simulink library "halout"  (R2021b)
settings: Solver=VariableStepAuto  StartTime=0.0  StopTime=10.0  RelTol=1e-3
undefined symbols (not defined in the file): C_TASK_5MS_S, FALSE, KHAL_CAN1FDAPS3E2E_flg, KHAL_CAN1FDAPS3TxReq_flg, KHAL_CAN1FDVCU2E2E_flg, KHAL_CAN1FDVCU2TxReq_flg, KHAL_CAN1FDVCU3E2E_flg, KHAL_CAN1FDVCU3TxReq_flg, KHAL_CAN1TxReq_flg, KHAL_CAN2TxReq_flg, KHAL_CAN3FDVCU1TxReq_flg, KHAL_CAN3FDVCU2E2E_flg, KHAL_CAN3FDVCU2TxReq_flg, KHAL_CAN3TxReq_flg, KHAL_CAN4FDVCU1E2E_flg, KHAL_CAN4FDVCU1TxReq_flg, KHAL_CAN4TxReq_flg, KHAL_CAN5TxReq_flg, ONE_INT, TRUE, ZERO_INT
libraries: FVT_lib x383, simulink x179
(part 8 of 20)

== system halout/HAL_OUT/CAN4/FD_DKC1_0x253 ==
  BSCP_outputs : Inport  OutDataTypeStr=Bus: BSCP_outputs
  BOUTP_outputs : Inport  Port=2  OutDataTypeStr=Bus: BOUTP_outputs
  ApproachUnlockSW : Subsystem
  BrkPedalPos : Subsystem
  BrkPedalPosSta : Subsystem
  BrkSwSta : Subsystem
  BrkSwV : Subsystem
  DSEATantiset : Subsystem
  DSEATentryfunset : Subsystem
  DSEATventreq : Subsystem
  FDCBCMATCtrlCmd : Subsystem
  FDCBCMLockAlarmCmd : Subsystem
  FDCBCMOutModeCmd : Subsystem
  FDCTHCMACTInitialCmd : Subsystem
  Ground1 : Ground
  HeadLampSW : Subsystem
  HoodLatchSW : Subsystem
  IVIISAOffsetSpd : Subsystem
  IVILocatedSTA : Subsystem
  IVIPTGModeSW : Subsystem
  IVIPTGOpenHeight : Subsystem
  IVIPTGStaSW : Subsystem
  IVIPTGUSStaSW : Subsystem
  IVITimeCheck : Subsystem
  IVITimeDay : Subsystem
  IVITimeHour : Subsystem
  IVITimeMinute : Subsystem
  IVITimeMonth : Subsystem
  IVITimeSecond : Subsystem
  IVITimeYear : Subsystem
  LDrvCtrlCmd : Subsystem
  LPasCtrlCmd : Subsystem
  LRLDCtrlCmd : Subsystem
  LRRDCtrlCmd : Subsystem
  MCPressure : Subsystem
  MCPressureV : Subsystem
  OFFACMODE : Subsystem
  PSEATventreq : Subsystem
  PTGInnerSW2 : Subsystem
  SenstivityPosition : Subsystem
  TurnSwTimeSet : Subsystem
  WalkawayLockSW : Subsystem
  bus_creator : BusCreator  Inputs=39  OutDataTypeStr=Bus: DT_CAN4_SG_FD_DKC1  NonVirtualBus=on
  bus_selector : BusSelector  OutputSignals=VSCP_CAN4FDDKC1ApproachUnlockSW_flg
  bus_selector1 : BusSelector  OutputSignals=VSCP_CAN4FDDKC1BrkPedalPos_pct
  bus_selector10 : BusSelector  OutputSignals=VSCP_CAN4FDDKC1HeadLampSW_enum
  bus_selector11 : BusSelector  OutputSignals=VSCP_CAN4FDDKC1HoodLatchSW_enum
  bus_selector12 : BusSelector  OutputSignals=VSCP_CAN4FDDKC1IVIISAOffsetSpd_enum
  bus_selector13 : BusSelector  OutputSignals=VSCP_CAN4FDDKC1IVILocatedSTA_enum
  bus_selector14 : BusSelector  OutputSignals=VSCP_CAN4FDDKC1IVIPTGModeSW_enum
  bus_selector15 : BusSelector  OutputSignals=VSCP_CAN4FDDKC1IVIPTGOpenHeight_enum
  bus_selector16 : BusSelector  OutputSignals=VSCP_CAN4FDDKC1IVIPTGStaSW_enum
  bus_selector17 : BusSelector  OutputSignals=VSCP_CAN4FDDKC1IVIPTGUSStaSW_flg
  bus_selector18 : BusSelector  OutputSignals=VSCP_CAN4FDDKC1IVITimeCheck_enum
  bus_selector19 : BusSelector  OutputSignals=VSCP_CAN4FDDKC1IVITimeDay_DAY
  bus_selector2 : BusSelector  OutputSignals=VSCP_CAN4FDDKC1BrkPedalPosSta_flg
  bus_selector20 : BusSelector  OutputSignals=VSCP_CAN4FDDKC1IVITimeHour_hr
  bus_selector21 : BusSelector  OutputSignals=VSCP_CAN4FDDKC1IVITimeMinute_min
  bus_selector22 : BusSelector  OutputSignals=VSCP_CAN4FDDKC1IVITimeMonth_MONTH
  bus_selector23 : BusSelector  OutputSignals=VSCP_CAN4FDDKC1IVITimeSecond_s
  bus_selector24 : BusSelector  OutputSignals=VSCP_CAN4FDDKC1IVITimeYear_YEAR
  bus_selector25 : BusSelector  OutputSignals=VOUTP_LDrvCtrlCmd_pct
  bus_selector26 : BusSelector  OutputSignals=VOUTP_LPasCtrlCmd_pct
  bus_selector27 : BusSelector  OutputSignals=VOUTP_LRLDCtrlCmd_pct
  bus_selector28 : BusSelector  OutputSignals=VOUTP_LRRDCtrlCmd_pct
  bus_selector29 : BusSelector  OutputSignals=VSCP_CAN4FDDKC1MCPressure_bar
  bus_selector3 : BusSelector  OutputSignals=VSCP_CAN4FDDKC1BrkSwSta_flg
  bus_selector30 : BusSelector  OutputSignals=VSCP_CAN4FDDKC1MCPressureV_flg
  bus_selector31 : BusSelector  OutputSignals=VSCP_CAN4FDDKC1OFFACMODE_enum
  bus_selector32 : BusSelector  OutputSignals=VSCP_CAN4FDDKC1PSEATventreq_enum
  bus_selector33 : BusSelector  OutputSignals=VOUTP_PTGInnerSW2_enum
  bus_selector34 : BusSelector  OutputSignals=VSCP_CAN4FDDKC1SenstivityPosition_enum
  bus_selector35 : BusSelector  OutputSignals=VSCP_CAN4FDDKC1TurnSwTimeSet_enum
  bus_selector36 : BusSelector  OutputSignals=VSCP_CAN4FDDKC1WalkawayLockSW_flg
  bus_selector37 : BusSelector  OutputSignals=VOUTP_OutMode_enum
  bus_selector4 : BusSelector  OutputSignals=VSCP_CAN4FDDKC1BrkSwV_flg
  bus_selector5 : BusSelector  OutputSignals=VSCP_CAN4FDDKC1DSEATantiset_flg
  bus_selector6 : BusSelector  OutputSignals=VSCP_CAN4FDDKC1DSEATentryfunset_flg
  bus_selector7 : BusSelector  OutputSignals=VSCP_CAN4FDDKC1DSEATventreq_enum
  bus_selector8 : BusSelector  OutputSignals=VOUTP_ATCtrl_enum
  bus_selector9 : BusSelector  OutputSignals=VOUTP_LockAlarm_enum
  FD_DKC1 : Outport
  wires:
  BSCP_outputs/1 -> [BSCP_outputs]
  BOUTP_outputs/1 -> [BOUTP_outputs]
  [CAN4_Approach_Unlock_SW] -> bus_creator/1  "CAN4_Approach_Unlock_SW"
  [CAN4_BrkPedalPos] -> bus_creator/2  "CAN4_BrkPedalPos"
  [CAN4_BrkPedalPos_Sta] -> bus_creator/3  "CAN4_BrkPedalPos_Sta"
  [CAN4_BrkSw_Sta] -> bus_creator/4  "CAN4_BrkSw_Sta"
  [CAN4_BrkSw_V] -> bus_creator/5  "CAN4_BrkSw_V"
  [CAN4_DSEAT_anti_set] -> bus_creator/6  "CAN4_DSEAT_anti_set"
  [CAN4_DSEAT_entryfun_set] -> bus_creator/7  "CAN4_DSEAT_entryfun_set"
  [CAN4_DSEAT_vent_req] -> bus_creator/8  "CAN4_DSEAT_vent_req"
  [CAN4_FDC_BCM_ATCtrl_Cmd] -> bus_creator/9  "CAN4_FDC_BCM_ATCtrl_Cmd"
  [CAN4_FDC_BCM_LockAlarm_Cmd] -> bus_creator/10  "CAN4_FDC_BCM_LockAlarm_Cmd"
  [CAN4_FDC_BCM_OutMode_Cmd] -> bus_creator/11  "CAN4_FDC_BCM_OutMode_Cmd"
  [CAN4_FDC_THCM_ACTInitial_Cmd] -> bus_creator/12  "CAN4_FDC_THCM_ACTInitial_Cmd"
  [CAN4_HeadLampSW] -> bus_creator/13  "CAN4_HeadLampSW"
  [CAN4_Hood_Latch_SW] -> bus_creator/14  "CAN4_Hood_Latch_SW"
  [CAN4_IVI_ISA_OffsetSpd] -> bus_creator/15  "CAN4_IVI_ISA_OffsetSpd"
  [CAN4_IVI_Located_STA] -> bus_creator/16  "CAN4_IVI_Located_STA"
  [CAN4_IVI_PTG_Mode_SW] -> bus_creator/17  "CAN4_IVI_PTG_Mode_SW"
  [CAN4_IVI_PTG_Open_Height] -> bus_creator/18  "CAN4_IVI_PTG_Open_Height"
  [CAN4_IVI_PTG_Sta_SW] -> bus_creator/19  "CAN4_IVI_PTG_Sta_SW"
  [CAN4_IVI_PTG_USSta_SW] -> bus_creator/20  "CAN4_IVI_PTG_USSta_SW"
  [CAN4_IVI_Time_Check] -> bus_creator/21  "CAN4_IVI_Time_Check"
  [CAN4_IVI_Time_Day] -> bus_creator/22  "CAN4_IVI_Time_Day"
  [CAN4_IVI_Time_Hour] -> bus_creator/23  "CAN4_IVI_Time_Hour"
  [CAN4_IVI_Time_Minute] -> bus_creator/24  "CAN4_IVI_Time_Minute"
  [CAN4_IVI_Time_Month] -> bus_creator/25  "CAN4_IVI_Time_Month"
  [CAN4_IVI_Time_Second] -> bus_creator/26  "CAN4_IVI_Time_Second"
  [CAN4_IVI_Time_Year] -> bus_creator/27  "CAN4_IVI_Time_Year"
  [CAN4_L_Drv_CtrlCmd] -> bus_creator/28  "CAN4_L_Drv_CtrlCmd"
  [CAN4_L_Pas_CtrlCmd] -> bus_creator/29  "CAN4_L_Pas_CtrlCmd"
  [CAN4_L_RLD_CtrlCmd] -> bus_creator/30  "CAN4_L_RLD_CtrlCmd"
  [CAN4_L_RRD_CtrlCmd] -> bus_creator/31  "CAN4_L_RRD_CtrlCmd"
  [CAN4_MCPressure] -> bus_creator/32  "CAN4_MCPressure"
  [CAN4_MCPressure_V] -> bus_creator/33  "CAN4_MCPressure_V"
  [CAN4_OFF_AC_MODE] -> bus_creator/34  "CAN4_OFF_AC_MODE"
  [CAN4_PSEAT_vent_req] -> bus_creator/35  "CAN4_PSEAT_vent_req"
  [CAN4_PTG_Inner_SW2] -> bus_creator/36  "CAN4_PTG_Inner_SW2"
  [CAN4_SenstivityPosition] -> bus_creator/37  "CAN4_SenstivityPosition"
  [CAN4_TurnSwTimeSet] -> bus_creator/38  "CAN4_TurnSwTimeSet"
  [CAN4_Walkaway_Lock_SW] -> bus_creator/39  "CAN4_Walkaway_Lock_SW"
  bus_creator/1 -> FD_DKC1/1
  ApproachUnlockSW/1(CAN4_Approach_Unlock_SW) -> [CAN4_Approach_Unlock_SW]
  BrkPedalPos/1(CAN4_BrkPedalPos) -> [CAN4_BrkPedalPos]
  BrkPedalPosSta/1(CAN4_BrkPedalPos_Sta) -> [CAN4_BrkPedalPos_Sta]
  BrkSwSta/1(CAN4_BrkSw_Sta) -> [CAN4_BrkSw_Sta]
  BrkSwV/1(CAN4_BrkSw_V) -> [CAN4_BrkSw_V]
  DSEATantiset/1(CAN4_DSEAT_anti_set) -> [CAN4_DSEAT_anti_set]
  DSEATentryfunset/1(CAN4_DSEAT_entryfun_set) -> [CAN4_DSEAT_entryfun_set]
  DSEATventreq/1(CAN4_DSEAT_vent_req) -> [CAN4_DSEAT_vent_req]
  FDCBCMATCtrlCmd/1(CAN4_FDC_BCM_ATCtrl_Cmd) -> [CAN4_FDC_BCM_ATCtrl_Cmd]
  FDCBCMLockAlarmCmd/1(CAN4_FDC_BCM_LockAlarm_Cmd) -> [CAN4_FDC_BCM_LockAlarm_Cmd]
  FDCBCMOutModeCmd/1(CAN4_FDC_BCM_OutMode_Cmd) -> [CAN4_FDC_BCM_OutMode_Cmd]
  FDCTHCMACTInitialCmd/1(CAN4_FDC_THCM_ACTInitial_Cmd) -> [CAN4_FDC_THCM_ACTInitial_Cmd]
  HeadLampSW/1(CAN4_HeadLampSW) -> [CAN4_HeadLampSW]
  HoodLatchSW/1(CAN4_Hood_Latch_SW) -> [CAN4_Hood_Latch_SW]
  IVIISAOffsetSpd/1(CAN4_IVI_ISA_OffsetSpd) -> [CAN4_IVI_ISA_OffsetSpd]
  IVILocatedSTA/1(CAN4_IVI_Located_STA) -> [CAN4_IVI_Located_STA]
  IVIPTGModeSW/1(CAN4_IVI_PTG_Mode_SW) -> [CAN4_IVI_PTG_Mode_SW]
  IVIPTGOpenHeight/1(CAN4_IVI_PTG_Open_Height) -> [CAN4_IVI_PTG_Open_Height]
  IVIPTGStaSW/1(CAN4_IVI_PTG_Sta_SW) -> [CAN4_IVI_PTG_Sta_SW]
  IVIPTGUSStaSW/1(CAN4_IVI_PTG_USSta_SW) -> [CAN4_IVI_PTG_USSta_SW]
  IVITimeCheck/1(CAN4_IVI_Time_Check) -> [CAN4_IVI_Time_Check]
  IVITimeDay/1(CAN4_IVI_Time_Day) -> [CAN4_IVI_Time_Day]
  IVITimeHour/1(CAN4_IVI_Time_Hour) -> [CAN4_IVI_Time_Hour]
  IVITimeMinute/1(CAN4_IVI_Time_Minute) -> [CAN4_IVI_Time_Minute]
  IVITimeMonth/1(CAN4_IVI_Time_Month) -> [CAN4_IVI_Time_Month]
  IVITimeSecond/1(CAN4_IVI_Time_Second) -> [CAN4_IVI_Time_Second]
  IVITimeYear/1(CAN4_IVI_Time_Year) -> [CAN4_IVI_Time_Year]
  LDrvCtrlCmd/1(CAN4_L_Drv_CtrlCmd) -> [CAN4_L_Drv_CtrlCmd]
  LPasCtrlCmd/1(CAN4_L_Pas_CtrlCmd) -> [CAN4_L_Pas_CtrlCmd]
  LRLDCtrlCmd/1(CAN4_L_RLD_CtrlCmd) -> [CAN4_L_RLD_CtrlCmd]
  LRRDCtrlCmd/1(CAN4_L_RRD_CtrlCmd) -> [CAN4_L_RRD_CtrlCmd]
  MCPressure/1(CAN4_MCPressure) -> [CAN4_MCPressure]
  MCPressureV/1(CAN4_MCPressure_V) -> [CAN4_MCPressure_V]
  OFFACMODE/1(CAN4_OFF_AC_MODE) -> [CAN4_OFF_AC_MODE]
  PSEATventreq/1(CAN4_PSEAT_vent_req) -> [CAN4_PSEAT_vent_req]
  PTGInnerSW2/1(CAN4_PTG_Inner_SW2) -> [CAN4_PTG_Inner_SW2]
  SenstivityPosition/1(CAN4_SenstivityPosition) -> [CAN4_SenstivityPosition]
  TurnSwTimeSet/1(CAN4_TurnSwTimeSet) -> [CAN4_TurnSwTimeSet]
  WalkawayLockSW/1(CAN4_Walkaway_Lock_SW) -> [CAN4_Walkaway_Lock_SW]
  bus_selector/1 -> ApproachUnlockSW/1(ApproachUnlockSW)  "<VSCP_CAN4FDDKC1ApproachUnlockSW_flg>"
  [BSCP_outputs] -> bus_selector/1
  bus_selector1/1 -> BrkPedalPos/1(BrkPedalPos)  "<VSCP_CAN4FDDKC1BrkPedalPos_pct>"
  [BSCP_outputs] -> bus_selector1/1
  bus_selector2/1 -> BrkPedalPosSta/1(BrkPedalPosSta)  "<VSCP_CAN4FDDKC1BrkPedalPosSta_flg>"
  [BSCP_outputs] -> bus_selector2/1
  bus_selector3/1 -> BrkSwSta/1(BrkSwSta)  "<VSCP_CAN4FDDKC1BrkSwSta_flg>"
  [BSCP_outputs] -> bus_selector3/1
  bus_selector4/1 -> BrkSwV/1(BrkSwV)  "<VSCP_CAN4FDDKC1BrkSwV_flg>"
  [BSCP_outputs] -> bus_selector4/1
  bus_selector5/1 -> DSEATantiset/1(DSEATantiset)  "<VSCP_CAN4FDDKC1DSEATantiset_flg>"
  [BSCP_outputs] -> bus_selector5/1
  bus_selector6/1 -> DSEATentryfunset/1(DSEATentryfunset)  "<VSCP_CAN4FDDKC1DSEATentryfunset_flg>"
  [BSCP_outputs] -> bus_selector6/1
  bus_selector7/1 -> DSEATventreq/1(DSEATventreq)  "<VSCP_CAN4FDDKC1DSEATventreq_enum>"
  [BSCP_outputs] -> bus_selector7/1
  bus_selector8/1 -> FDCBCMATCtrlCmd/1(FDCBCMATCtrlCmd)  "<VOUTP_ATCtrl_enum>"
  [BOUTP_outputs] -> bus_selector8/1
  bus_selector9/1 -> FDCBCMLockAlarmCmd/1(FDCBCMLockAlarmCmd)  "<VOUTP_LockAlarm_enum>"
  [BOUTP_outputs] -> bus_selector9/1
  Ground1/1 -> FDCTHCMACTInitialCmd/1(FDCTHCMACTInitialCmd)
  bus_selector10/1 -> HeadLampSW/1(HeadLampSW)  "<VSCP_CAN4FDDKC1HeadLampSW_enum>"
  [BSCP_outputs] -> bus_selector10/1
  bus_selector11/1 -> HoodLatchSW/1(HoodLatchSW)  "<VSCP_CAN4FDDKC1HoodLatchSW_enum>"
  [BSCP_outputs] -> bus_selector11/1
  bus_selector12/1 -> IVIISAOffsetSpd/1(IVIISAOffsetSpd)  "<VSCP_CAN4FDDKC1IVIISAOffsetSpd_enum>"
  [BSCP_outputs] -> bus_selector12/1
  bus_selector13/1 -> IVILocatedSTA/1(IVILocatedSTA)  "<VSCP_CAN4FDDKC1IVILocatedSTA_enum>"
  [BSCP_outputs] -> bus_selector13/1
  bus_selector14/1 -> IVIPTGModeSW/1(IVIPTGModeSW)  "<VSCP_CAN4FDDKC1IVIPTGModeSW_enum>"
  [BSCP_outputs] -> bus_selector14/1
  bus_selector15/1 -> IVIPTGOpenHeight/1(IVIPTGOpenHeight)  "<VSCP_CAN4FDDKC1IVIPTGOpenHeight_enum>"
  [BSCP_outputs] -> bus_selector15/1
  bus_selector16/1 -> IVIPTGStaSW/1(IVIPTGStaSW)  "<VSCP_CAN4FDDKC1IVIPTGStaSW_enum>"
  [BSCP_outputs] -> bus_selector16/1
  bus_selector17/1 -> IVIPTGUSStaSW/1(IVIPTGUSStaSW)  "<VSCP_CAN4FDDKC1IVIPTGUSStaSW_flg>"
  [BSCP_outputs] -> bus_selector17/1
  bus_selector18/1 -> IVITimeCheck/1(IVITimeCheck)  "<VSCP_CAN4FDDKC1IVITimeCheck_enum>"
  [BSCP_outputs] -> bus_selector18/1
  bus_selector19/1 -> IVITimeDay/1(IVITimeDay)  "<VSCP_CAN4FDDKC1IVITimeDay_DAY>"
  [BSCP_outputs] -> bus_selector19/1
  bus_selector20/1 -> IVITimeHour/1(IVITimeHour)  "<VSCP_CAN4FDDKC1IVITimeHour_hr>"
  [BSCP_outputs] -> bus_selector20/1
  bus_selector21/1 -> IVITimeMinute/1(IVITimeMinute)  "<VSCP_CAN4FDDKC1IVITimeMinute_min>"
  [BSCP_outputs] -> bus_selector21/1
  bus_selector22/1 -> IVITimeMonth/1(IVITimeMonth)  "<VSCP_CAN4FDDKC1IVITimeMonth_MONTH>"
  [BSCP_outputs] -> bus_selector22/1
  bus_selector23/1 -> IVITimeSecond/1(IVITimeSecond)  "<VSCP_CAN4FDDKC1IVITimeSecond_s>"
  [BSCP_outputs] -> bus_selector23/1
  bus_selector24/1 -> IVITimeYear/1(IVITimeYear)  "<VSCP_CAN4FDDKC1IVITimeYear_YEAR>"
  [BSCP_outputs] -> bus_selector24/1
  bus_selector25/1 -> LDrvCtrlCmd/1(LDrvCtrlCmd)  "<VOUTP_LDrvCtrlCmd_pct>"
  [BOUTP_outputs] -> bus_selector25/1
  bus_selector26/1 -> LPasCtrlCmd/1(LPasCtrlCmd)  "<VOUTP_LPasCtrlCmd_pct>"
  [BOUTP_outputs] -> bus_selector26/1
  bus_selector27/1 -> LRLDCtrlCmd/1(LRLDCtrlCmd)  "<VOUTP_LRLDCtrlCmd_pct>"
  [BOUTP_outputs] -> bus_selector27/1
  bus_selector28/1 -> LRRDCtrlCmd/1(LRRDCtrlCmd)  "<VOUTP_LRRDCtrlCmd_pct>"
  [BOUTP_outputs] -> bus_selector28/1
  bus_selector29/1 -> MCPressure/1(MCPressure)  "<VSCP_CAN4FDDKC1MCPressure_bar>"
  [BSCP_outputs] -> bus_selector29/1
  bus_selector30/1 -> MCPressureV/1(MCPressureV)  "<VSCP_CAN4FDDKC1MCPressureV_flg>"
  [BSCP_outputs] -> bus_selector30/1
  bus_selector31/1 -> OFFACMODE/1(OFFACMODE)  "<VSCP_CAN4FDDKC1OFFACMODE_enum>"
  [BSCP_outputs] -> bus_selector31/1
  bus_selector32/1 -> PSEATventreq/1(PSEATventreq)  "<VSCP_CAN4FDDKC1PSEATventreq_enum>"
  [BSCP_outputs] -> bus_selector32/1
  bus_selector33/1 -> PTGInnerSW2/1(PTGInnerSW2)  "<VOUTP_PTGInnerSW2_enum>"
  [BOUTP_outputs] -> bus_selector33/1
  bus_selector34/1 -> SenstivityPosition/1(SenstivityPosition)  "<VSCP_CAN4FDDKC1SenstivityPosition_enum>"
  [BSCP_outputs] -> bus_selector34/1
  bus_selector35/1 -> TurnSwTimeSet/1(TurnSwTimeSet)  "<VSCP_CAN4FDDKC1TurnSwTimeSet_enum>"
  [BSCP_outputs] -> bus_selector35/1
  bus_selector36/1 -> WalkawayLockSW/1(WalkawayLockSW)  "<VSCP_CAN4FDDKC1WalkawayLockSW_flg>"
  [BSCP_outputs] -> bus_selector36/1
  [BOUTP_outputs] -> bus_selector37/1
  bus_selector37/1 -> FDCBCMOutModeCmd/1(FDCBCMOutModeCmd)  "<VOUTP_OutMode_enum>"

== system halout/HAL_OUT/CAN4/FD_THCM1_0x182 ==
  BSCP_outputs : Inport  OutDataTypeStr=Bus: BSCP_outputs
  BOUTP_outputs : Inport  Port=2  OutDataTypeStr=Bus: BOUTP_outputs
  BatteryMode : Subsystem
  CCUACLampSts : Subsystem
  CCUACMaxLampSts : Subsystem
  CCUAutoLampSts : Subsystem
  CCUAutoMidLampSts : Subsystem
  CCUDispalyRequest : Subsystem
  CCUEcoSts : Subsystem
  CCUFrtOnOffLampSts : Subsystem
  CCUHEATMaxLampSts : Subsystem
  CCURrOnOffLampSts : Subsystem
  CCUSyncLampSts : Subsystem
  CabinMode : Subsystem
  EDriveMode : Subsystem
  FDAGSCmd : Subsystem
  FDRecyAutoCmd : Subsystem
  FrCoolantflow : Subsystem
  FrCoolanttemp : Subsystem
  Ground{,1..17} (18 alike) : Ground
  HPThermalRecoveryReq : Subsystem
  RrCoolantflow : Subsystem
  RrCoolanttemp : Subsystem
  bus_creator : BusCreator  Inputs=37  OutDataTypeStr=Bus: DT_CAN4_SG_FD_THCM1  NonVirtualBus=on
  bus_selector : BusSelector  OutputSignals=VOUTP_BatteryMode_enum
  bus_selector1 : BusSelector  OutputSignals=VOUTP_CCUACLampSts_flg
  bus_selector10 : BusSelector  OutputSignals=VOUTP_sigAmbAirT_C
  bus_selector11 : BusSelector  OutputSignals=VOUTP_sigCbnAirT_C
  bus_selector12 : BusSelector  OutputSignals=VOUTP_sigCbnSolarLeft_W
  bus_selector13 : BusSelector  OutputSignals=VOUTP_sigCbnSolarRight_W
  bus_selector14 : BusSelector  OutputSignals=VOUTP_sigClntTHvBattOut_C
  bus_selector15 : BusSelector  OutputSignals=VOUTP_sigRecircSt_flg
  bus_selector16 : BusSelector  OutputSignals=VOUTP_sigSetTempZon1St_C
  bus_selector17 : BusSelector  OutputSignals=VOUTP_sigSetTempZon2St_C
  bus_selector18 : BusSelector  OutputSignals=VOUTP_sigWindDirZon1St_enum
  bus_selector2 : BusSelector  OutputSignals=VOUTP_CCUACMaxLampSts_flg
  bus_selector3 : BusSelector  OutputSignals=VOUTP_CCUAutoLampSts_flg
  bus_selector4 : BusSelector  OutputSignals=VOUTP_CCUSyncLampSts_flg
  bus_selector5 : BusSelector  OutputSignals=VOUTP_CabinMode_enum
  bus_selector6 : BusSelector  OutputSignals=VOUTP_EDriveMode_enum
  bus_selector7 : BusSelector  OutputSignals=VOUTP_FDAGSCmd_enum
  bus_selector8 : BusSelector  OutputSignals=VOUTP_FDRecyAutoCmd_enum
  bus_selector9 : BusSelector  OutputSignals=VOUTP_sigAirIntenZon1St_enum
  sigAirIntenZon1St : Subsystem
  sigAirIntenZon3St : Subsystem
  sigAmbAirT : Subsystem
  sigCbnAirT : Subsystem
  sigCbnPTCPwrAct : Subsystem
  sigCbnSolarLeft : Subsystem
  sigCbnSolarRight : Subsystem
  sigClmtCmprPwrAct : Subsystem
  sigClntTHvBattOut : Subsystem
  sigDfrstSt : Subsystem
  sigHvacSt : Subsystem
  sigRecircSt : Subsystem
  sigSetTempZon1St : Subsystem
  sigSetTempZon2St : Subsystem
  sigSetTempZon3St : Subsystem
  sigWindDirZon1St : Subsystem
  sigWindDirZon3St : Subsystem
  FD_THCM1 : Outport
  wires:
  BSCP_outputs/1 -> [BSCP_outputs]
  BOUTP_outputs/1 -> [BOUTP_outputs]
  [CAN4_BatteryMode] -> bus_creator/1  "CAN4_BatteryMode"
  [CAN4_CCU_ACLampSts] -> bus_creator/2  "CAN4_CCU_ACLampSts"
  [CAN4_CCU_ACMaxLampSts] -> bus_creator/3  "CAN4_CCU_ACMaxLampSts"
  [CAN4_CCU_AutoLampSts] -> bus_creator/4  "CAN4_CCU_AutoLampSts"
  [CAN4_CCU_AutoMidLampSts] -> bus_creator/5  "CAN4_CCU_AutoMidLampSts"
  [CAN4_CCU_Dispaly_Request] -> bus_creator/6  "CAN4_CCU_Dispaly_Request"
  [CAN4_CCU_EcoSts] -> bus_creator/7  "CAN4_CCU_EcoSts"
  [CAN4_CCU_FrtOnOffLampSts] -> bus_creator/8  "CAN4_CCU_FrtOnOffLampSts"
  [CAN4_CCU_HEATMaxLampSts] -> bus_creator/9  "CAN4_CCU_HEATMaxLampSts"
  [CAN4_CCU_RrOnOffLampSts] -> bus_creator/10  "CAN4_CCU_RrOnOffLampSts"
  [CAN4_CCU_SyncLampSts] -> bus_creator/11  "CAN4_CCU_SyncLampSts"
  [CAN4_CabinMode] -> bus_creator/12  "CAN4_CabinMode"
  [CAN4_EDriveMode] -> bus_creator/13  "CAN4_EDriveMode"
  [CAN4_FD_AGS_Cmd] -> bus_creator/14  "CAN4_FD_AGS_Cmd"
  [CAN4_FD_RecyAuto_Cmd] -> bus_creator/15  "CAN4_FD_RecyAuto_Cmd"
  [CAN4_Fr_Coolantflow] -> bus_creator/16  "CAN4_Fr_Coolantflow"
  [CAN4_Fr_Coolanttemp] -> bus_creator/17  "CAN4_Fr_Coolanttemp"
  [CAN4_HPThermalRecoveryReq] -> bus_creator/18  "CAN4_HPThermalRecoveryReq"
  [CAN4_Rr_Coolantflow] -> bus_creator/19  "CAN4_Rr_Coolantflow"
  [CAN4_Rr_Coolanttemp] -> bus_creator/20  "CAN4_Rr_Coolanttemp"
  [CAN4_sigAirIntenZon1St] -> bus_creator/21  "CAN4_sigAirIntenZon1St"
  [CAN4_sigAirIntenZon3St] -> bus_creator/22  "CAN4_sigAirIntenZon3St"
  [CAN4_sigAmbAirT] -> bus_creator/23  "CAN4_sigAmbAirT"
  [CAN4_sigCbnAirT] -> bus_creator/24  "CAN4_sigCbnAirT"
  [CAN4_sigCbnPTCPwrAct] -> bus_creator/25  "CAN4_sigCbnPTCPwrAct"
  [CAN4_sigCbnSolarLeft] -> bus_creator/26  "CAN4_sigCbnSolarLeft"
  [CAN4_sigCbnSolarRight] -> bus_creator/27  "CAN4_sigCbnSolarRight"
  [CAN4_sigClmtCmprPwrAct] -> bus_creator/28  "CAN4_sigClmtCmprPwrAct"
  [CAN4_sigClntTHvBattOut] -> bus_creator/29  "CAN4_sigClntTHvBattOut"
  [CAN4_sigDfrstSt] -> bus_creator/30  "CAN4_sigDfrstSt"
  [CAN4_sigHvacSt] -> bus_creator/31  "CAN4_sigHvacSt"
  [CAN4_sigRecircSt] -> bus_creator/32  "CAN4_sigRecircSt"
  [CAN4_sigSetTempZon1St] -> bus_creator/33  "CAN4_sigSetTempZon1St"
  [CAN4_sigSetTempZon2St] -> bus_creator/34  "CAN4_sigSetTempZon2St"
  [CAN4_sigSetTempZon3St] -> bus_creator/35  "CAN4_sigSetTempZon3St"
  [CAN4_sigWindDirZon1St] -> bus_creator/36  "CAN4_sigWindDirZon1St"
  [CAN4_sigWindDirZon3St] -> bus_creator/37  "CAN4_sigWindDirZon3St"
  bus_creator/1 -> FD_THCM1/1
  BatteryMode/1(CAN4_BatteryMode) -> [CAN4_BatteryMode]
  CCUACLampSts/1(CAN4_CCU_ACLampSts) -> [CAN4_CCU_ACLampSts]
  CCUACMaxLampSts/1(CAN4_CCU_ACMaxLampSts) -> [CAN4_CCU_ACMaxLampSts]
  CCUAutoLampSts/1(CAN4_CCU_AutoLampSts) -> [CAN4_CCU_AutoLampSts]
  CCUAutoMidLampSts/1(CAN4_CCU_AutoMidLampSts) -> [CAN4_CCU_AutoMidLampSts]
  CCUDispalyRequest/1(CAN4_CCU_Dispaly_Request) -> [CAN4_CCU_Dispaly_Request]
  CCUEcoSts/1(CAN4_CCU_EcoSts) -> [CAN4_CCU_EcoSts]
  CCUFrtOnOffLampSts/1(CAN4_CCU_FrtOnOffLampSts) -> [CAN4_CCU_FrtOnOffLampSts]
  CCUHEATMaxLampSts/1(CAN4_CCU_HEATMaxLampSts) -> [CAN4_CCU_HEATMaxLampSts]
  CCURrOnOffLampSts/1(CAN4_CCU_RrOnOffLampSts) -> [CAN4_CCU_RrOnOffLampSts]
  CCUSyncLampSts/1(CAN4_CCU_SyncLampSts) -> [CAN4_CCU_SyncLampSts]
  CabinMode/1(CAN4_CabinMode) -> [CAN4_CabinMode]
  EDriveMode/1(CAN4_EDriveMode) -> [CAN4_EDriveMode]
  FDAGSCmd/1(CAN4_FD_AGS_Cmd) -> [CAN4_FD_AGS_Cmd]
  FDRecyAutoCmd/1(CAN4_FD_RecyAuto_Cmd) -> [CAN4_FD_RecyAuto_Cmd]
  FrCoolantflow/1(CAN4_Fr_Coolantflow) -> [CAN4_Fr_Coolantflow]
  FrCoolanttemp/1(CAN4_Fr_Coolanttemp) -> [CAN4_Fr_Coolanttemp]
  HPThermalRecoveryReq/1(CAN4_HPThermalRecoveryReq) -> [CAN4_HPThermalRecoveryReq]
  RrCoolantflow/1(CAN4_Rr_Coolantflow) -> [CAN4_Rr_Coolantflow]
  RrCoolanttemp/1(CAN4_Rr_Coolanttemp) -> [CAN4_Rr_Coolanttemp]
  sigAirIntenZon1St/1(CAN4_sigAirIntenZon1St) -> [CAN4_sigAirIntenZon1St]
  sigAirIntenZon3St/1(CAN4_sigAirIntenZon3St) -> [CAN4_sigAirIntenZon3St]
  sigAmbAirT/1(CAN4_sigAmbAirT) -> [CAN4_sigAmbAirT]
  sigCbnAirT/1(CAN4_sigCbnAirT) -> [CAN4_sigCbnAirT]
  sigCbnPTCPwrAct/1(CAN4_sigCbnPTCPwrAct) -> [CAN4_sigCbnPTCPwrAct]
  sigCbnSolarLeft/1(CAN4_sigCbnSolarLeft) -> [CAN4_sigCbnSolarLeft]
  sigCbnSolarRight/1(CAN4_sigCbnSolarRight) -> [CAN4_sigCbnSolarRight]
  sigClmtCmprPwrAct/1(CAN4_sigClmtCmprPwrAct) -> [CAN4_sigClmtCmprPwrAct]
  sigClntTHvBattOut/1(CAN4_sigClntTHvBattOut) -> [CAN4_sigClntTHvBattOut]
  sigDfrstSt/1(CAN4_sigDfrstSt) -> [CAN4_sigDfrstSt]
  sigHvacSt/1(CAN4_sigHvacSt) -> [CAN4_sigHvacSt]
  sigRecircSt/1(CAN4_sigRecircSt) -> [CAN4_sigRecircSt]
  sigSetTempZon1St/1(CAN4_sigSetTempZon1St) -> [CAN4_sigSetTempZon1St]
  sigSetTempZon2St/1(CAN4_sigSetTempZon2St) -> [CAN4_sigSetTempZon2St]
  sigSetTempZon3St/1(CAN4_sigSetTempZon3St) -> [CAN4_sigSetTempZon3St]
  sigWindDirZon1St/1(CAN4_sigWindDirZon1St) -> [CAN4_sigWindDirZon1St]
  sigWindDirZon3St/1(CAN4_sigWindDirZon3St) -> [CAN4_sigWindDirZon3St]
  bus_selector/1 -> BatteryMode/1(BatteryMode)  "<VOUTP_BatteryMode_enum>"
  [BOUTP_outputs] -> bus_selector/1
  bus_selector1/1 -> CCUACLampSts/1(CCUACLampSts)  "<VOUTP_CCUACLampSts_flg>"
  [BOUTP_outputs] -> bus_selector1/1
  bus_selector2/1 -> CCUACMaxLampSts/1(CCUACMaxLampSts)  "<VOUTP_CCUACMaxLampSts_flg>"
  [BOUTP_outputs] -> bus_selector2/1
  bus_selector3/1 -> CCUAutoLampSts/1(CCUAutoLampSts)  "<VOUTP_CCUAutoLampSts_flg>"
  [BOUTP_outputs] -> bus_selector3/1
  Ground/1 -> CCUAutoMidLampSts/1(CCUAutoMidLampSts)
  Ground1/1 -> CCUDispalyRequest/1(CCUDispalyRequest)
  Ground2/1 -> CCUEcoSts/1(CCUEcoSts)
  Ground3/1 -> CCUFrtOnOffLampSts/1(CCUFrtOnOffLampSts)
  Ground4/1 -> CCUHEATMaxLampSts/1(CCUHEATMaxLampSts)
  Ground5/1 -> CCURrOnOffLampSts/1(CCURrOnOffLampSts)
  bus_selector4/1 -> CCUSyncLampSts/1(CCUSyncLampSts)  "<VOUTP_CCUSyncLampSts_flg>"
  [BOUTP_outputs] -> bus_selector4/1
  bus_selector5/1 -> CabinMode/1(CabinMode)  "<VOUTP_CabinMode_enum>"
  [BOUTP_outputs] -> bus_selector5/1
  bus_selector6/1 -> EDriveMode/1(EDriveMode)  "<VOUTP_EDriveMode_enum>"
  [BOUTP_outputs] -> bus_selector6/1
  bus_selector7/1 -> FDAGSCmd/1(FDAGSCmd)  "<VOUTP_FDAGSCmd_enum>"
  [BOUTP_outputs] -> bus_selector7/1
  bus_selector8/1 -> FDRecyAutoCmd/1(FDRecyAutoCmd)  "<VOUTP_FDRecyAutoCmd_enum>"
  [BOUTP_outputs] -> bus_selector8/1
  Ground6/1 -> FrCoolantflow/1(FrCoolantflow)
  Ground7/1 -> FrCoolanttemp/1(FrCoolanttemp)
  Ground8/1 -> HPThermalRecoveryReq/1(HPThermalRecoveryReq)
  Ground9/1 -> RrCoolantflow/1(RrCoolantflow)
  Ground10/1 -> RrCoolanttemp/1(RrCoolanttemp)
  bus_selector9/1 -> sigAirIntenZon1St/1(sigAirIntenZon1St)  "<VOUTP_sigAirIntenZon1St_enum>"
  [BOUTP_outputs] -> bus_selector9/1
  Ground11/1 -> sigAirIntenZon3St/1(sigAirIntenZon3St)
  bus_selector10/1 -> sigAmbAirT/1(sigAmbAirT)  "<VOUTP_sigAmbAirT_C>"
  [BOUTP_outputs] -> bus_selector10/1
  bus_selector11/1 -> sigCbnAirT/1(sigCbnAirT)  "<VOUTP_sigCbnAirT_C>"
  [BOUTP_outputs] -> bus_selector11/1
  Ground12/1 -> sigCbnPTCPwrAct/1(sigCbnPTCPwrAct)
  bus_selector12/1 -> sigCbnSolarLeft/1(sigCbnSolarLeft)  "<VOUTP_sigCbnSolarLeft_W>"
  [BOUTP_outputs] -> bus_selector12/1
  bus_selector13/1 -> sigCbnSolarRight/1(sigCbnSolarRight)  "<VOUTP_sigCbnSolarRight_W>"
  [BOUTP_outputs] -> bus_selector13/1
  Ground13/1 -> sigClmtCmprPwrAct/1(sigClmtCmprPwrAct)
  bus_selector14/1 -> sigClntTHvBattOut/1(sigClntTHvBattOut)  "<VOUTP_sigClntTHvBattOut_C>"
  [BOUTP_outputs] -> bus_selector14/1
  Ground14/1 -> sigDfrstSt/1(sigDfrstSt)
  Ground15/1 -> sigHvacSt/1(sigHvacSt)
  bus_selector15/1 -> sigRecircSt/1(sigRecircSt)  "<VOUTP_sigRecircSt_flg>"
  [BOUTP_outputs] -> bus_selector15/1
  bus_selector16/1 -> sigSetTempZon1St/1(sigSetTempZon1St)  "<VOUTP_sigSetTempZon1St_C>"
  [BOUTP_outputs] -> bus_selector16/1
  bus_selector17/1 -> sigSetTempZon2St/1(sigSetTempZon2St)  "<VOUTP_sigSetTempZon2St_C>"
  [BOUTP_outputs] -> bus_selector17/1
  Ground16/1 -> sigSetTempZon3St/1(sigSetTempZon3St)
  bus_selector18/1 -> sigWindDirZon1St/1(sigWindDirZon1St)  "<VOUTP_sigWindDirZon1St_enum>"
  [BOUTP_outputs] -> bus_selector18/1
  Ground17/1 -> sigWindDirZon3St/1(sigWindDirZon3St)

== system halout/HAL_OUT/CAN4/FD_THCM2_0x186 ==
  BSCP_outputs : Inport  OutDataTypeStr=Bus: BSCP_outputs
  BOUTP_outputs : Inport  Port=2  OutDataTypeStr=Bus: BOUTP_outputs
  ACSubMode : Subsystem
  APTCActFrRiPwr : Subsystem
  BatLoopActWtFlw : Subsystem
  CCUCbnPreACWkSts : Subsystem
  CCUCbnPreEstimdTi : Subsystem
  CCUCbnPreSts : Subsystem
  CCUHiVoltageReq : Subsystem
  CoolgFanActDuty : Subsystem
  DeiceModReq : Subsystem
  FDBlowerCmd : Subsystem
  FDCompCmd : Subsystem
  FDEWP1Cmd : Subsystem
  FDEWP2Cmd : Subsystem
  FDEWP3Cmd : Subsystem
  FDEXV1Cmd : Subsystem
  FDEXV2Cmd : Subsystem
  FDFWVCmd : Subsystem
  FDFrLeAPTCHeatPwrCmd : Subsystem
  FDFrRiAPTCHeatPwrCmd : Subsystem
  FDFrWPTCHeatPwrCmd : Subsystem
  FDRrAPTCHeatPwrCmd : Subsystem
  FDSOTXVCmd : Subsystem
  FDSOV1Cmd : Subsystem
  FDSOV2Cmd : Subsystem
  FDSOV3Cmd : Subsystem
  FDTWVCmd : Subsystem
  Ground{,1..6} (7 alike) : Ground
  bus_creator : BusCreator  Inputs=26  OutDataTypeStr=Bus: DT_CAN4_SG_FD_THCM2  NonVirtualBus=on
  bus_selector : BusSelector  OutputSignals=VOUTP_ACSubMode_enum
  bus_selector1 : BusSelector  OutputSignals=VOUTP_CoolgFanActDuty_pct
  bus_selector10 : BusSelector  OutputSignals=VOUTP_FDFrLeAPTCHeatPwrCmd_W
  bus_selector11 : BusSelector  OutputSignals=VOUTP_FDFrRiAPTCHeatPwrCmd_W
  bus_selector12 : BusSelector  OutputSignals=VOUTP_FDFrWPTCHeatPwrCmd_W
  bus_selector13 : BusSelector  OutputSignals=VOUTP_FDRrAPTCHeatPwrCmd_W
  bus_selector14 : BusSelector  OutputSignals=VOUTP_FDSOTXVCmd_flg
  bus_selector15 : BusSelector  OutputSignals=VOUTP_FDSOV1Cmd_flg
  bus_selector16 : BusSelector  OutputSignals=VOUTP_FDSOV2Cmd_flg
  bus_selector17 : BusSelector  OutputSignals=VOUTP_FDSOV3Cmd_flg
  bus_selector18 : BusSelector  OutputSignals=VOUTP_FDTWVCmd_pct
  bus_selector2 : BusSelector  OutputSignals=VOUTP_FDBlowerCmd_pct
  bus_selector3 : BusSelector  OutputSignals=VOUTP_FDCompCmd_rpm
  bus_selector4 : BusSelector  OutputSignals=VOUTP_FDEWP1Cmd_enum
  bus_selector5 : BusSelector  OutputSignals=VOUTP_FDEWP2Cmd_enum
  bus_selector6 : BusSelector  OutputSignals=VOUTP_FDEWP3Cmd_enum
  bus_selector7 : BusSelector  OutputSignals=VOUTP_FDEXV1Cmd_step
  bus_selector8 : BusSelector  OutputSignals=VOUTP_FDEXV2Cmd_step
  bus_selector9 : BusSelector  OutputSignals=VOUTP_FDFWVCmd_flg
  FD_THCM2 : Outport
  wires:
  BSCP_outputs/1 -> [BSCP_outputs]
  BOUTP_outputs/1 -> [BOUTP_outputs]
  [CAN4_ACSubMode] -> bus_creator/1  "CAN4_ACSubMode"
  [CAN4_APTC_ActFrRiPwr] -> bus_creator/2  "CAN4_APTC_ActFrRiPwr"
  [CAN4_BatLoopActWtFlw] -> bus_creator/3  "CAN4_BatLoopActWtFlw"
  [CAN4_CCU_CbnPreACWkSts] -> bus_creator/4  "CAN4_CCU_CbnPreACWkSts"
  [CAN4_CCU_CbnPreEstimdTi] -> bus_creator/5  "CAN4_CCU_CbnPreEstimdTi"
  [CAN4_CCU_CbnPreSts] -> bus_creator/6  "CAN4_CCU_CbnPreSts"
  [CAN4_CCU_HiVoltageReq] -> bus_creator/7  "CAN4_CCU_HiVoltageReq"
  [CAN4_CoolgFanActDuty] -> bus_creator/8  "CAN4_CoolgFanActDuty"
  [CAN4_DeiceModReq] -> bus_creator/9  "CAN4_DeiceModReq"
  [CAN4_FD_Blower_Cmd] -> bus_creator/10  "CAN4_FD_Blower_Cmd"
  [CAN4_FD_Comp_Cmd] -> bus_creator/11  "CAN4_FD_Comp_Cmd"
  [CAN4_FD_EWP1_Cmd] -> bus_creator/12  "CAN4_FD_EWP1_Cmd"
  [CAN4_FD_EWP2_Cmd] -> bus_creator/13  "CAN4_FD_EWP2_Cmd"
  [CAN4_FD_EWP3_Cmd] -> bus_creator/14  "CAN4_FD_EWP3_Cmd"
  [CAN4_FD_EXV1_Cmd] -> bus_creator/15  "CAN4_FD_EXV1_Cmd"
  [CAN4_FD_EXV2_Cmd] -> bus_creator/16  "CAN4_FD_EXV2_Cmd"
  [CAN4_FD_FWV_Cmd] -> bus_creator/17  "CAN4_FD_FWV_Cmd"
  [CAN4_FD_FrLeAPTCHeatPwr_Cmd] -> bus_creator/18  "CAN4_FD_FrLeAPTCHeatPwr_Cmd"
  [CAN4_FD_FrRiAPTCHeatPwr_Cmd] -> bus_creator/19  "CAN4_FD_FrRiAPTCHeatPwr_Cmd"
  [CAN4_FD_FrWPTCHeatPwr_Cmd] -> bus_creator/20  "CAN4_FD_FrWPTCHeatPwr_Cmd"
  [CAN4_FD_RrAPTCHeatPwr_Cmd] -> bus_creator/21  "CAN4_FD_RrAPTCHeatPwr_Cmd"
  [CAN4_FD_SOTXV_Cmd] -> bus_creator/22  "CAN4_FD_SOTXV_Cmd"
  [CAN4_FD_SOV1_Cmd] -> bus_creator/23  "CAN4_FD_SOV1_Cmd"
  [CAN4_FD_SOV2_Cmd] -> bus_creator/24  "CAN4_FD_SOV2_Cmd"
  [CAN4_FD_SOV3_Cmd] -> bus_creator/25  "CAN4_FD_SOV3_Cmd"
  [CAN4_FD_TWV_Cmd] -> bus_creator/26  "CAN4_FD_TWV_Cmd"
  bus_creator/1 -> FD_THCM2/1
  ACSubMode/1(CAN4_ACSubMode) -> [CAN4_ACSubMode]
  APTCActFrRiPwr/1(CAN4_APTC_ActFrRiPwr) -> [CAN4_APTC_ActFrRiPwr]
  BatLoopActWtFlw/1(CAN4_BatLoopActWtFlw) -> [CAN4_BatLoopActWtFlw]
  CCUCbnPreACWkSts/1(CAN4_CCU_CbnPreACWkSts) -> [CAN4_CCU_CbnPreACWkSts]
  CCUCbnPreEstimdTi/1(CAN4_CCU_CbnPreEstimdTi) -> [CAN4_CCU_CbnPreEstimdTi]
  CCUCbnPreSts/1(CAN4_CCU_CbnPreSts) -> [CAN4_CCU_CbnPreSts]
  CCUHiVoltageReq/1(CAN4_CCU_HiVoltageReq) -> [CAN4_CCU_HiVoltageReq]
  CoolgFanActDuty/1(CAN4_CoolgFanActDuty) -> [CAN4_CoolgFanActDuty]
  DeiceModReq/1(CAN4_DeiceModReq) -> [CAN4_DeiceModReq]
  FDBlowerCmd/1(CAN4_FD_Blower_Cmd) -> [CAN4_FD_Blower_Cmd]
  FDCompCmd/1(CAN4_FD_Comp_Cmd) -> [CAN4_FD_Comp_Cmd]
  FDEWP1Cmd/1(CAN4_FD_EWP1_Cmd) -> [CAN4_FD_EWP1_Cmd]
  FDEWP2Cmd/1(CAN4_FD_EWP2_Cmd) -> [CAN4_FD_EWP2_Cmd]
  FDEWP3Cmd/1(CAN4_FD_EWP3_Cmd) -> [CAN4_FD_EWP3_Cmd]
  FDEXV1Cmd/1(CAN4_FD_EXV1_Cmd) -> [CAN4_FD_EXV1_Cmd]
  FDEXV2Cmd/1(CAN4_FD_EXV2_Cmd) -> [CAN4_FD_EXV2_Cmd]
  FDFWVCmd/1(CAN4_FD_FWV_Cmd) -> [CAN4_FD_FWV_Cmd]
  FDFrLeAPTCHeatPwrCmd/1(CAN4_FD_FrLeAPTCHeatPwr_Cmd) -> [CAN4_FD_FrLeAPTCHeatPwr_Cmd]
  FDFrRiAPTCHeatPwrCmd/1(CAN4_FD_FrRiAPTCHeatPwr_Cmd) -> [CAN4_FD_FrRiAPTCHeatPwr_Cmd]
  FDFrWPTCHeatPwrCmd/1(CAN4_FD_FrWPTCHeatPwr_Cmd) -> [CAN4_FD_FrWPTCHeatPwr_Cmd]
  FDRrAPTCHeatPwrCmd/1(CAN4_FD_RrAPTCHeatPwr_Cmd) -> [CAN4_FD_RrAPTCHeatPwr_Cmd]
  FDSOTXVCmd/1(CAN4_FD_SOTXV_Cmd) -> [CAN4_FD_SOTXV_Cmd]
  FDSOV1Cmd/1(CAN4_FD_SOV1_Cmd) -> [CAN4_FD_SOV1_Cmd]
  FDSOV2Cmd/1(CAN4_FD_SOV2_Cmd) -> [CAN4_FD_SOV2_Cmd]
  FDSOV3Cmd/1(CAN4_FD_SOV3_Cmd) -> [CAN4_FD_SOV3_Cmd]
  FDTWVCmd/1(CAN4_FD_TWV_Cmd) -> [CAN4_FD_TWV_Cmd]
  bus_selector/1 -> ACSubMode/1(ACSubMode)  "<VOUTP_ACSubMode_enum>"
  [BOUTP_outputs] -> bus_selector/1
  Ground/1 -> APTCActFrRiPwr/1(APTCActFrRiPwr)
  Ground1/1 -> BatLoopActWtFlw/1(BatLoopActWtFlw)
  Ground2/1 -> CCUCbnPreACWkSts/1(CCUCbnPreACWkSts)
  Ground3/1 -> CCUCbnPreEstimdTi/1(CCUCbnPreEstimdTi)
  Ground4/1 -> CCUCbnPreSts/1(CCUCbnPreSts)
  Ground5/1 -> CCUHiVoltageReq/1(CCUHiVoltageReq)
  bus_selector1/1 -> CoolgFanActDuty/1(CoolgFanActDuty)  "<VOUTP_CoolgFanActDuty_pct>"
  [BOUTP_outputs] -> bus_selector1/1
  Ground6/1 -> DeiceModReq/1(DeiceModReq)
  bus_selector2/1 -> FDBlowerCmd/1(FDBlowerCmd)  "<VOUTP_FDBlowerCmd_pct>"
  [BOUTP_outputs] -> bus_selector2/1
  bus_selector3/1 -> FDCompCmd/1(FDCompCmd)  "<VOUTP_FDCompCmd_rpm>"
  [BOUTP_outputs] -> bus_selector3/1
  bus_selector4/1 -> FDEWP1Cmd/1(FDEWP1Cmd)  "<VOUTP_FDEWP1Cmd_enum>"
  [BOUTP_outputs] -> bus_selector4/1
  bus_selector5/1 -> FDEWP2Cmd/1(FDEWP2Cmd)  "<VOUTP_FDEWP2Cmd_enum>"
  [BOUTP_outputs] -> bus_selector5/1
  bus_selector6/1 -> FDEWP3Cmd/1(FDEWP3Cmd)  "<VOUTP_FDEWP3Cmd_enum>"
  [BOUTP_outputs] -> bus_selector6/1
  bus_selector7/1 -> FDEXV1Cmd/1(FDEXV1Cmd)  "<VOUTP_FDEXV1Cmd_step>"
  [BOUTP_outputs] -> bus_selector7/1
  bus_selector8/1 -> FDEXV2Cmd/1(FDEXV2Cmd)  "<VOUTP_FDEXV2Cmd_step>"
  [BOUTP_outputs] -> bus_selector8/1
  bus_selector9/1 -> FDFWVCmd/1(FDFWVCmd)  "<VOUTP_FDFWVCmd_flg>"
  [BOUTP_outputs] -> bus_selector9/1
  bus_selector10/1 -> FDFrLeAPTCHeatPwrCmd/1(FDFrLeAPTCHeatPwrCmd)  "<VOUTP_FDFrLeAPTCHeatPwrCmd_W>"
  [BOUTP_outputs] -> bus_selector10/1
  bus_selector11/1 -> FDFrRiAPTCHeatPwrCmd/1(FDFrRiAPTCHeatPwrCmd)  "<VOUTP_FDFrRiAPTCHeatPwrCmd_W>"
  [BOUTP_outputs] -> bus_selector11/1
  bus_selector12/1 -> FDFrWPTCHeatPwrCmd/1(FDFrWPTCHeatPwrCmd)  "<VOUTP_FDFrWPTCHeatPwrCmd_W>"
  [BOUTP_outputs] -> bus_selector12/1
  bus_selector13/1 -> FDRrAPTCHeatPwrCmd/1(FDRrAPTCHeatPwrCmd)  "<VOUTP_FDRrAPTCHeatPwrCmd_W>"
  [BOUTP_outputs] -> bus_selector13/1
  bus_selector14/1 -> FDSOTXVCmd/1(FDSOTXVCmd)  "<VOUTP_FDSOTXVCmd_flg>"
  [BOUTP_outputs] -> bus_selector14/1
  bus_selector15/1 -> FDSOV1Cmd/1(FDSOV1Cmd)  "<VOUTP_FDSOV1Cmd_flg>"
  [BOUTP_outputs] -> bus_selector15/1
  bus_selector16/1 -> FDSOV2Cmd/1(FDSOV2Cmd)  "<VOUTP_FDSOV2Cmd_flg>"
  [BOUTP_outputs] -> bus_selector16/1
  bus_selector17/1 -> FDSOV3Cmd/1(FDSOV3Cmd)  "<VOUTP_FDSOV3Cmd_flg>"
  [BOUTP_outputs] -> bus_selector17/1
  bus_selector18/1 -> FDTWVCmd/1(FDTWVCmd)  "<VOUTP_FDTWVCmd_pct>"
  [BOUTP_outputs] -> bus_selector18/1
